simulink model "DFT_Ex3"  (R2023a)
settings: Solver=VariableStepAuto  StartTime=0.0  StopTime=0.5  RelTol=1e-3
undefined symbols (not defined in the file): None, S, vsva2197, xcvc1902
libraries: dspsrcs4 x2, aieDSP x1, vmcUtilities x1
settings Model: Creator=sdegala  LastModifiedBy=robg
settings ModelReferenceCC: EnableRefExpFcnMdlSchedulingChecks=on

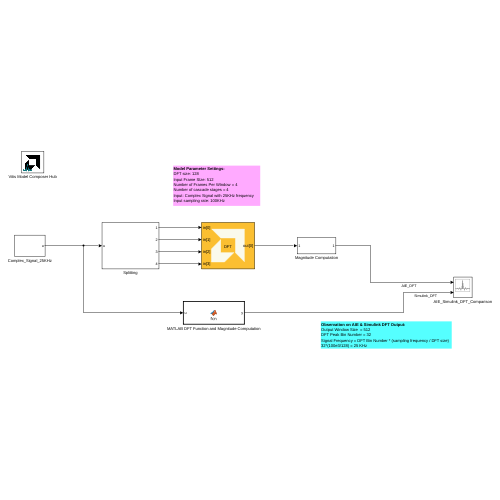
[thumbnail: Simulink's stored preview of the top-level diagram]
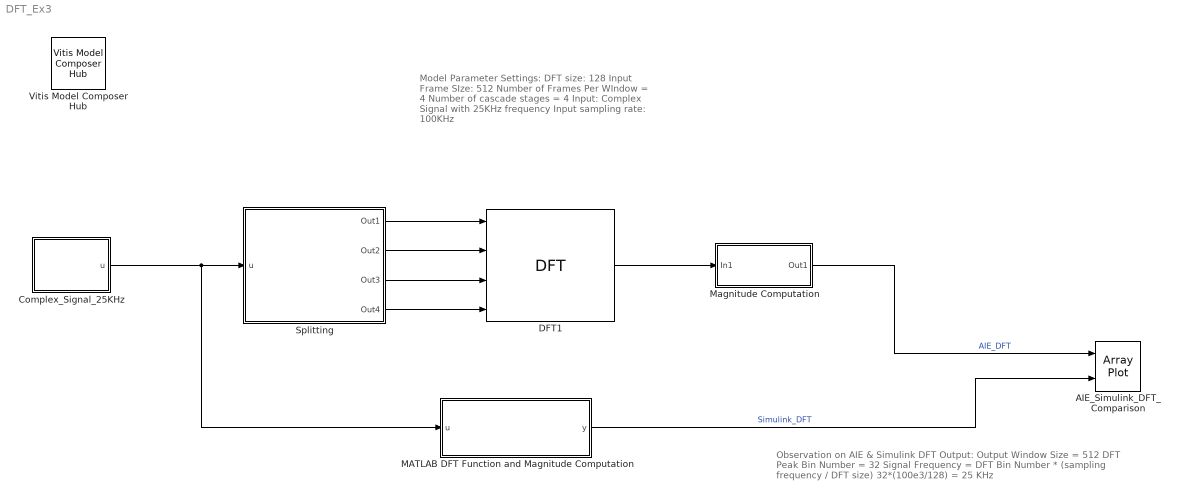
== system DFT_Ex3 ==
  note: Model Parameter Settings:
      | DFT size: 128
      | Input Frame SIze: 512
      | Number of Frames Per WIndow = 4
      | Number of cascade stages = 4
      | Input: Complex Signal with 25KHz frequency
      | Input sampling rate: 100KHz
  note: Observation on AIE & Simulink DFT Output:
      | Output Window Size = 512
      | DFT Peak Bin Number = 32
      | Signal Frequency = DFT Bin Number * (sampling frequency / DFT size)
      | 32*(100e3/128) = 25 KHz
  AIE_Simulink_DFT_Comparison : ArrayPlot  NumInputPorts=2  WindowPosition=[2.000000,26.000000,1280.000000,749.000000,]  Visible=on  ScopeFrameLocation=window  YLimits=[-24 216]  ShowLegend=on
  Complex_Signal_25KHz : Subsystem
  DFT1 : aieDSP/DFT  data_type=cint16  twiddle_type=cint16  point_size=128  num_frames=4  shift_val=0  rnd_mode=Round symmetrical to infinity  ssr=1  sat_mode=0-None  casc_length=4  AIE_VARIANT=1  blockJsonConstraints=[]  blockJsonConstraintsInternal=[]  spec=vmc_dft.json  SerializedMaskParamNames=[]  SerializedMaskParamValues=[]  SerializedMaskParamVisibilities=[]  block_type=DFT  SerializedMaskParamDataypes=typename|typename|uint|uint|uint|uint|uint|uint|uint|uint  SerializedMaskParamEnumStrArr=0|0|0|0|0|Floor,Ceiling,Round to positive infinity,Round to negative infinity,Round symmetrical to infinity,Round symmetrical to zero,Round convergent to even,Round convergent to odd|0|0-None,1-Asymmetric,3-Symmetric|0|0  SerializedMaskParamEnumValArr=0|0|0|0|0|0,1,2,3,4,5,6,7|0|0,1,3|0|0  SerializedMaskParamVectorArr=0|0|0|0|0|0|0|0|0|0
  MATLAB DFT Function and Magnitude Computation : MATLAB Function  TreatAsAtomicUnit=on
  Magnitude Computation : Subsystem
  Splitting : Subsystem
  Vitis Model Composer Hub : vmcUtilities/Vitis Model Composer Hub  Tag=genX  CodeGeneration=off  StartColumn=1  NumberOfColumns=1  TargetDirectory=./code  exportDesign=off  analyzeDesign=off  validateDesignOnHw=off  ExportType=AI Engines  IpVendor=xilinx.com  IpLibrary=hls  IpVersion=1.0  IpHWLanguage=Verilog  AieCompilerOptions={}  AieSimulatorOptions={}  CreateTestbench=off  TestbenchStackSize=10  RunRtlSim=off  RunCSim=off  RunAieSim=off  AieSimTimeout=50000  RunAieSimProfiling=off  LaunchVitisAnalyzer=off  PlotOutput=off  RunX86Sim=off  X86SimTimeout=10  GenHwImage=off  GenLibadfXo=off  GenHwValidationCode=off  PlatformType=Not Specified  HwSystemType=Baremetal  HwValidationTarget=hw  ProjDevice=xcvc1902-vsva2197-1LP-e-S  ProjDevicePart=xcvc1902-vsva2197-1LP-e-S  AIEType=AIE  SamplePeriod=-1  ClockFrequency=200  DataPathParallelism=1  xilinxfamily=versalaicore  part=xcvc1902  speed=-1LP-e-S  package=vsva2197  directory=./code  testbench=off  incr_netlist=off  synthesis_tool=Vivado  clock_wrapper=Clock Enables  dbl_ovrd=According to Block Masks  dcm_input_clock_period=10  sysclk_period=10  simulink_period=1  eval_field=0  LogFileName=''  NThreads=4
  wires:
  Complex_Signal_25KHz/1(u) -> MATLAB DFT Function and Magnitude Computation/1(u), Splitting/1(u)
  DFT1/1 -> Magnitude Computation/1(In1)
  Magnitude Computation/1(Out1) -> AIE_Simulink_DFT_Comparison/1  "AIE_DFT"
  MATLAB DFT Function and Magnitude Computation/1(y) -> AIE_Simulink_DFT_Comparison/2  "Simulink_DFT"
  Splitting/1(Out1) -> DFT1/1
  Splitting/2(Out2) -> DFT1/2
  Splitting/3(Out3) -> DFT1/3
  Splitting/4(Out4) -> DFT1/4

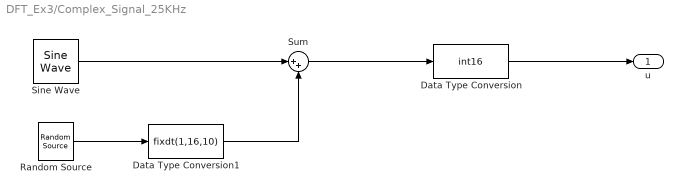
== system DFT_Ex3/Complex_Signal_25KHz ==
  Data Type Conversion : DataTypeConversion  OutDataTypeStr=int16  SaturateOnIntegerOverflow=off  RndMeth=Floor
  Data Type Conversion1 : DataTypeConversion  OutDataTypeStr=fixdt(1,16,10)  SaturateOnIntegerOverflow=off  RndMeth=Floor
  Random Source : dspsrcs4/Random Source  SrcType=Gaussian  NormMethod=Ziggurat  CltLength=12  MinVal=0  MaxVal=1  MeanVal=0  VarVal=0.5  RepMode=Not repeatable  rawSeed=1  IsInherit=off  SampMode=Discrete  SampTime=1/100e3  SampFrame=512  DataType=Single  OutComplex=Real  OutputFrames=off
  Sine Wave : dspsrcs4/Sine Wave  Amplitude=10  Frequency=25e3  Phase=0  SampleMode=Discrete  OutComplex=Complex  CompMethod=Table lookup  TableSize=Speed  SampleTime=1/100e3  SamplesPerFrame=512  ResetState=Restart at time zero  OutputFrames=off  dataType=Fixed-point  wordLen=16  udDataType=sfix(16)  fracBitsMode=User-defined  numFracBits=10  OutDataTypeStr=fixdt(1,16,10)  LastOutDataTypeStr=fixdt(1,16,10)
  Sum : Sum  Inputs=|++
  u : Outport
  wires:
  Sine Wave/1 -> Sum/1
  Data Type Conversion/1 -> u/1
  Random Source/1 -> Data Type Conversion1/1
  Sum/1 -> Data Type Conversion/1
  Data Type Conversion1/1 -> Sum/2

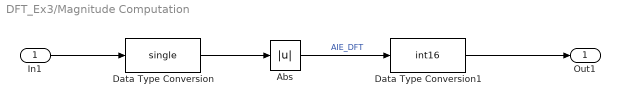
== system DFT_Ex3/Magnitude Computation ==
  In1 : Inport
  Abs : Abs  SaturateOnIntegerOverflow=off
  Data Type Conversion : DataTypeConversion  OutDataTypeStr=single  SaturateOnIntegerOverflow=off  RndMeth=Floor
  Data Type Conversion1 : DataTypeConversion  OutDataTypeStr=int16  SaturateOnIntegerOverflow=off  RndMeth=Floor
  Out1 : Outport
  wires:
  Data Type Conversion/1 -> Abs/1
  Data Type Conversion1/1 -> Out1/1
  Abs/1 -> Data Type Conversion1/1  "AIE_DFT"
  In1/1 -> Data Type Conversion/1

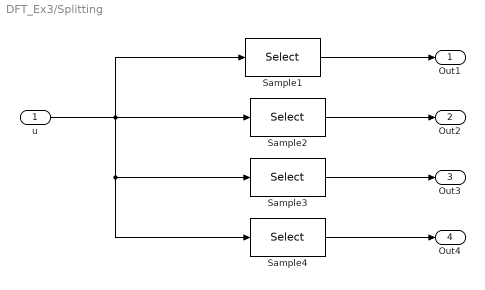
== system DFT_Ex3/Splitting ==
  u : Inport
  Sample1 : Selector  InputPortWidth=512  IndexOptions=Index vector (dialog)  Indices=1:4:512  OutputSizes=1
  Sample2 : Selector  InputPortWidth=512  IndexOptions=Index vector (dialog)  Indices=2:4:512  OutputSizes=1
  Sample3 : Selector  InputPortWidth=512  IndexOptions=Index vector (dialog)  Indices=3:4:512  OutputSizes=1
  Sample4 : Selector  InputPortWidth=512  IndexOptions=Index vector (dialog)  Indices=4:4:512  OutputSizes=1
  Out1 : Outport
  Out2 : Outport  Port=2
  Out3 : Outport  Port=3
  Out4 : Outport  Port=4
  wires:
  u/1 -> Sample4/1, Sample3/1, Sample2/1, Sample1/1
  Sample2/1 -> Out2/1
  Sample1/1 -> Out1/1
  Sample3/1 -> Out3/1
  Sample4/1 -> Out4/1

== matlab function DFT_Ex3/MATLAB DFT Function and Magnitude Computation ==
  data: u input; y output

function y = fcn(u)

DFT_Size = 128; % DFT Size
FramesPerWindow = 4; %No.of Frames Per Window
u = single(u);

X = single(complex(zeros(DFT_Size,FramesPerWindow)));

for m = 1:1:FramesPerWindow
for k = 0:DFT_Size-1
    for n = 0:DFT_Size-1
        X(k+1,m) = X(k+1,m) + u(n+1)*exp(-1i*2*pi*n*k/DFT_Size);
    end
end
end

y = int16(abs(reshape(X,DFT_Size*FramesPerWindow,1)));
